simulink model "MotorLabDemonstrationV2"  (R2022b)
settings: Solver=FixedStepAuto  StartTime=0.0  StopTime=Inf  RelTol=1e-3  EnableMultiTasking=on
libraries: arduinolib x10, arduinosensorlib x2
settings Model: SimulationMode=external  ExtModeTrigDuration=2  Creator=amanc  LastModifiedBy=amanc
settings SolverCC: AutoInsertRateTranBlk=on
settings OptimizationCC: EnhancedBackFolding=on  PassReuseOutputArgsAs=Individual arguments  ZeroExternalMemoryAtStartup=off  ZeroInternalMemoryAtStartup=off  MaxStackSize=64  OptimizeBlockOrder=speed  DifferentSizesBufferReuse=on  OptimizationCustomize=off  EfficientTunableParamExpr=on
settings DebuggingCC: ParameterTunabilityLossMsg=error
settings HardwareCC: ProdBitPerInt=16  ProdBitPerPointer=16  ProdBitPerSizeT=16  ProdBitPerPtrDiffT=16  ProdLargestAtomicFloat=None  ProdWordSize=8  ProdHWDeviceType=Atmel->AVR  UseEmbeddedCoderFeatures=off
settings SFSimCC: MATLABDynamicMemAlloc=off
settings RTWCC: Description=Embedded Coder  SystemTargetFile=ert.tlc  HardwareBoard=Arduino Mega 2560  TemplateMakefile=ert_default_tmf  Toolchain=Arduino AVR  BuildConfiguration=Faster Runs
settings CodeAppCC: ForceParamTrailComments=on  OperatorAnnotations=on  SimulinkDataObjDesc=on  SFDataObjDesc=on  InsertBlockDesc=on
settings ERTTargetCC: SupportContinuousTime=on  SupportNonInlinedSFcns=on  SupportVariableSizeSignals=on  ExtMode=on  ExtModeTransport=3  ExtModeStaticAlloc=on  ExtModeAutomaticAllocSize=off  ExtModeStaticAllocSize=2048  ExtModeMexFile=ext_xcp  ExtModeMexArgs=0 3 921600  ExtModeIntrfLevel=Level2 - Open  ERTSrcFileBannerTemplate=codertarget_code_template.cgt  ERTHdrFileBannerTemplate=codertarget_code_template.cgt  ERTDataSrcFileTemplate=codertarget_code_template.cgt  ERTDataHdrFileTemplate=codertarget_code_template.cgt

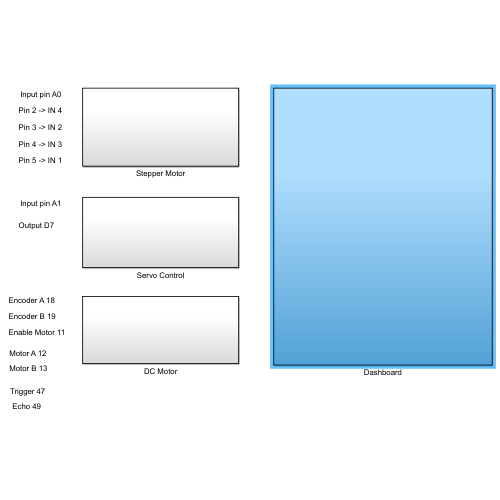
[thumbnail: Simulink's stored preview of the top-level diagram]
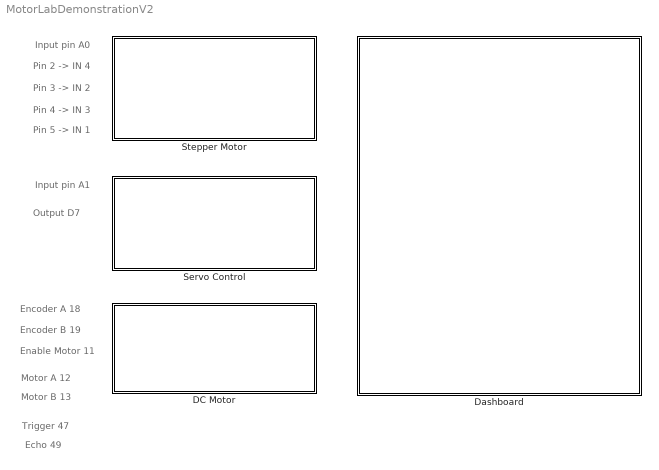
== system MotorLabDemonstrationV2 ==
  note: Echo 49
  note: Trigger 47
  note: Motor A 12
  note: Encoder A 18
  note: Pin 2 -> IN 4
  note: Input pin A0
  note: Pin 3 -> IN 2
  note: Pin 4 -> IN 3
  note: Pin 5 -> IN 1
  note: Output D7
  note: Input pin A1
  note: Encoder B 19
  note: Enable Motor 11
  note: Motor B 13
  DC Motor : Subsystem
  Dashboard : Subsystem
  Servo Control : Subsystem
  Stepper Motor : Subsystem

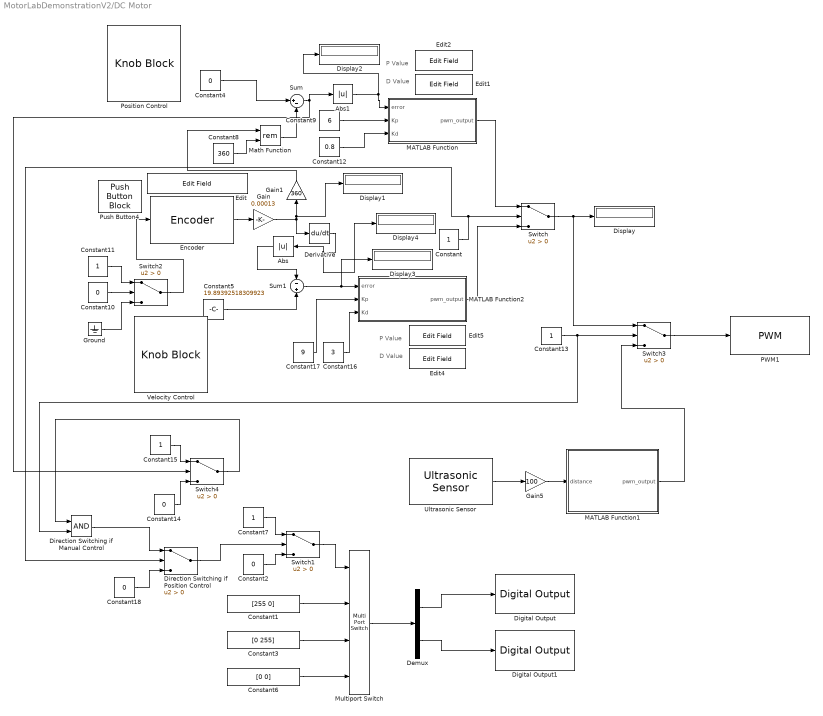
== system MotorLabDemonstrationV2/DC Motor ==
  note: P Value
  note: D Value
  note: P Value
  note: D Value
  Abs : Abs  SaturateOnIntegerOverflow=off
  Abs1 : Abs  SaturateOnIntegerOverflow=off
  Constant{,7,11,13,15} (5 alike) : Constant
  Constant1 : Constant  Value=[255 0]  OutDataTypeStr=uint8
  Constant{2,4,10,14,18} (5 alike) : Constant  Value=0
  Constant12 : Constant  Value=0.8
  Constant16 : Constant  Value=3
  Constant17 : Constant  Value=9
  Constant3 : Constant  Value=[0 255]  OutDataTypeStr=uint8
  Constant5 : Constant  Value=19.89392518309923
  Constant6 : Constant  Value=[0 0]  OutDataTypeStr=uint8
  Constant8 : Constant  Value=360
  Constant9 : Constant  Value=6
  Demux : Demux  Outputs=2
  Derivative : Derivative
  Digital Output : arduinolib/Digital Output  pinNumber=12  Direction=output  blockPlatform=arduino
  Digital Output1 : arduinolib/Digital Output  pinNumber=13  Direction=output  blockPlatform=arduino
  Direction Switching if Manual Control : Logic  AllPortsSameDT=off  OutDataTypeStr=boolean
  Direction Switching if Position Control : Switch  Criteria=u2 > Threshold  SaturateOnIntegerOverflow=off  InputSameDT=off
  Display{,1..4} (5 alike) : Display
  Edit{,1..2,4..5} (5 alike) : EditField  LabelPosition=Hide  ShowInitialText=on  Alignment=Center
  Encoder : arduinosensorlib/Encoder  InputA=18  InputB=19  Mode=Reset by external signal  SampleTime=-1
  Gain : Gain  Gain=0.00013  OutDataTypeStr=double
  Gain1 : Gain  Gain=360
  Gain5 : Gain  Gain=100
  Ground : Ground
  MATLAB Function : MATLAB Function  TreatAsAtomicUnit=on
  MATLAB Function1 : MATLAB Function  TreatAsAtomicUnit=on
  MATLAB Function2 : MATLAB Function  TreatAsAtomicUnit=on
  Math Function : Math  Operator=rem
  Multiport Switch : MultiPortSwitch  DataPortOrder=Zero-based contiguous  Inputs=2  DataPortForDefault=Additional data port  DiagnosticForDefault=None  zeroidx=on  SaturateOnIntegerOverflow=off
  PWM1 : arduinolib/PWM  pinNumber=11  frequencyType=Default  desiredFrequency=490.2  achievableFrequency=490.2
  Position Control : KnobBlock  LabelPosition=Hide  ScaleMax=360
  Push Button4 : PushButtonBlock  ButtonText=Reset  OffValue=0.000000
  Sum : Sum  Inputs=|+-
  Sum1 : Sum  Inputs=-|+
  Switch{,1..4} (5 alike) : Switch  Criteria=u2 > Threshold  SaturateOnIntegerOverflow=off  InputSameDT=off
  Ultrasonic Sensor : arduinosensorlib/Ultrasonic Sensor  NumSignalPins=2  TrigPin=47  EchoPin=49  SignalPin=3  SampleTime_=0.01  blockPlatform=ARDUINO
  Velocity Control : KnobBlock  LabelPosition=Hide  ScaleMax=20
  wires:
  Constant13/1 -> Direction Switching if Manual Control/2, Switch3/2
  MATLAB Function1/1(pwm_output) -> Switch3/3
  Constant10/1 -> Switch2/2
  Math Function/1 -> Sum/2
  Constant15/1 -> Switch4/1
  Constant11/1 -> Switch2/1
  MATLAB Function/1(pwm_output) -> Switch/1
  Gain/1 -> Display1/1, Gain1/1, Derivative/1
  MATLAB Function2/1(pwm_output) -> Switch/3
  Constant2/1 -> Switch1/3
  Gain1/1 -> Math Function/1
  Ground/1 -> Switch2/3
  Switch/1 -> Switch3/1, Display/1
  Constant17/1 -> MATLAB Function2/2(Kp)
  Sum1/1 -> Display3/1, MATLAB Function2/1(error)
  Constant12/1 -> MATLAB Function/3(Kd)
  Switch4/1 -> Direction Switching if Manual Control/1
  Constant9/1 -> MATLAB Function/2(Kp)
  Constant8/1 -> Math Function/2
  Constant5/1 -> Sum1/2
  Constant4/1 -> Sum/1
  Gain5/1 -> MATLAB Function1/1(distance)
  Constant7/1 -> Switch1/1
  Ultrasonic Sensor/1 -> Gain5/1
  Constant6/1 -> Multiport Switch/4
  Multiport Switch/1 -> Demux/1
  Constant16/1 -> MATLAB Function2/3(Kd)
  Encoder/1 -> Gain/1
  Constant1/1 -> Multiport Switch/2
  Demux/1 -> Digital Output/1
  Sum/1 -> Abs1/1, Switch4/2
  Switch1/1 -> Multiport Switch/1
  Constant14/1 -> Switch4/3
  Switch2/1 -> Encoder/1
  Constant3/1 -> Multiport Switch/3
  Constant/1 -> Direction Switching if Position Control/2, Switch/2
  Switch3/1 -> PWM1/1
  Demux/2 -> Digital Output1/1
  Constant18/1 -> Direction Switching if Position Control/3
  Direction Switching if Position Control/1 -> Switch1/2
  Direction Switching if Manual Control/1 -> Direction Switching if Position Control/1
  Derivative/1 -> Abs/1, Display4/1
  Abs/1 -> Sum1/1
  Abs1/1 -> MATLAB Function/1(error), Display2/1

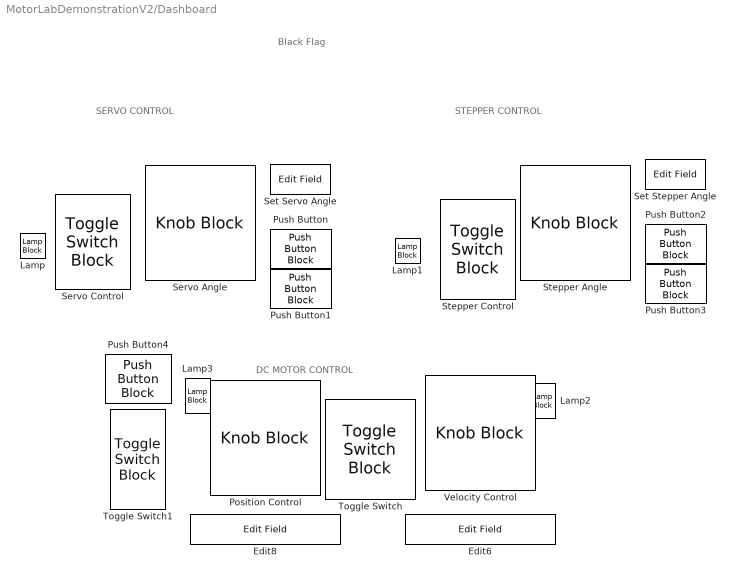
== system MotorLabDemonstrationV2/Dashboard ==
  note: Black Flag
  note: SERVO CONTROL
  note: STEPPER CONTROL
  note: DC MOTOR CONTROL
  Edit6 : EditField  LabelPosition=Hide  ShowInitialText=on  Alignment=Center
  Edit8 : EditField  LabelPosition=Hide  ShowInitialText=on  Alignment=Center
  Lamp{,1..3} (4 alike) : LampBlock  LabelPosition=Hide
  Position Control : KnobBlock  LabelPosition=Hide  ScaleMax=360
  Push Button : PushButtonBlock  ButtonText=Minimum  OnValue=0  ButtonType=Latch  OffValue=180.000000
  Push Button1 : PushButtonBlock  ButtonText=Maximum  OnValue=180  ButtonType=Latch  OffValue=0.000000
  Push Button2 : PushButtonBlock  ButtonText=Minimum  OnValue=-360  ButtonType=Latch  OffValue=0.000000
  Push Button3 : PushButtonBlock  ButtonText=Maximum  OnValue=360  ButtonType=Latch  OffValue=-360.000000
  Push Button4 : PushButtonBlock  ButtonText=Reset  OffValue=0.000000
  Servo Angle : KnobBlock  LabelPosition=Hide  ScaleMax=180
  Servo Control : ToggleSwitchBlock  LabelPosition=Hide
      settings: Values={{'Manual', 'Sensor Input'}, [0 1]}
  Set Servo Angle : EditField  LabelPosition=Hide  ShowInitialText=on  Alignment=Center
  Set Stepper Angle : EditField  LabelPosition=Hide  ShowInitialText=on  Alignment=Center
  Stepper Angle : KnobBlock  LabelPosition=Hide  ScaleMin=-360  ScaleMax=360
  Stepper Control : ToggleSwitchBlock  LabelPosition=Hide
      settings: Values={{'Manual', 'Sensor Control'}, [0 1]}
  Toggle Switch : ToggleSwitchBlock  LabelPosition=Hide
      settings: Values={{'Velocity Control', 'Position Control'}, [0 1]}
  Toggle Switch1 : ToggleSwitchBlock  LabelPosition=Hide
      settings: Values={{'Sensor', 'Manual'}, [0 1]}
  Velocity Control : KnobBlock  LabelPosition=Hide  ScaleMax=20

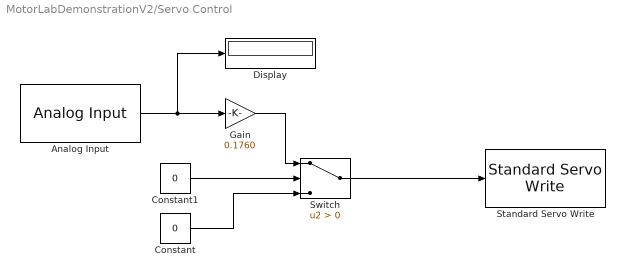
== system MotorLabDemonstrationV2/Servo Control ==
  Analog Input : arduinolib/Analog Input  pinNumber=2  ReadResultsOnly=off  ConversionTriggerSource=Software  ExternalTriggerType=uint32( 0 )  OutputDataType=uint16  EnableConversionCompleteNotify=off  EnableOuputStatus=off  SampleTime=0.01  blockPlatform=arduino
  Constant : Constant  Value=0  OutDataTypeStr=uint8
  Constant1 : Constant  Value=0
  Display : Display
  Gain : Gain  Gain=0.1760  OutDataTypeStr=uint8
  Standard Servo Write : arduinolib/Standard Servo Write  pinNumber=7  ServoIndex=0  blockPlatform=ARDUINO
  Switch : Switch  Criteria=u2 > Threshold  OutDataTypeStr=uint8  SaturateOnIntegerOverflow=off  InputSameDT=off
  wires:
  Analog Input/1 -> Display/1, Gain/1
  Constant1/1 -> Switch/2
  Switch/1 -> Standard Servo Write/1
  Gain/1 -> Switch/1
  Constant/1 -> Switch/3

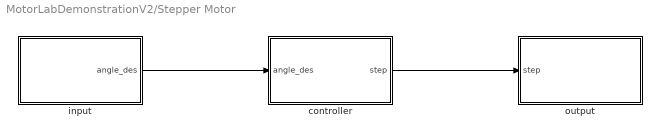
== system MotorLabDemonstrationV2/Stepper Motor ==
  controller : Subsystem
  input : Subsystem
  output : Subsystem
  wires:
  input/1(angle_des) -> controller/1(angle_des)
  controller/1(step) -> output/1(step)

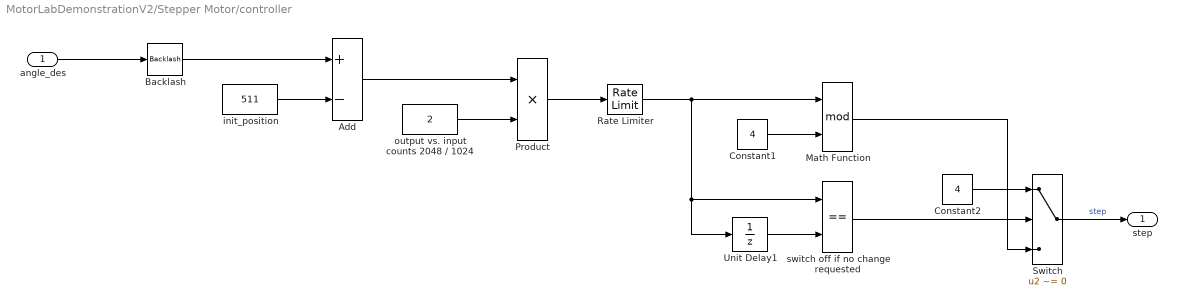
== system MotorLabDemonstrationV2/Stepper Motor/controller ==
  angle_des : Inport
  Add : Sum  Inputs=+-  InputSameDT=on
  Backlash : Backlash  BacklashWidth=6  InitialOutput=511
  Constant1 : Constant  Value=4  OutDataTypeStr=int16
  Constant2 : Constant  Value=4  OutDataTypeStr=int16
  Math Function : Math  Operator=mod  SignedPower=on  OutputSignalType=real
  Product : Product  InputSameDT=on  OutDataTypeStr=int16  RndMeth=Zero
  Rate Limiter : RateLimiter  RisingSlewLimit=100  FallingSlewLimit=-100  SampleTimeMode=inherited
  Switch : Switch  Criteria=u2 ~= 0  SaturateOnIntegerOverflow=off
  Unit Delay1 : UnitDelay  SampleTime=-1  HasFrameUpgradeWarning=on
  init_position : Constant  Value=511  OutDataTypeStr=int16
  output vs. input counts 2048 / 1024 : Constant  Value=2  OutDataTypeStr=int16
  switch off if no change requested : RelationalOperator  Operator===  OutDataTypeStr=boolean
  step : Outport
  wires:
  angle_des/1 -> Backlash/1
  init_position/1 -> Add/2
  Add/1 -> Product/1
  output vs. input counts 2048 / 1024/1 -> Product/2
  Product/1 -> Rate Limiter/1
  Constant1/1 -> Math Function/2
  Rate Limiter/1 -> switch off if no change requested/1, Unit Delay1/1, Math Function/1
  Backlash/1 -> Add/1
  Switch/1 -> step/1  "step"
  Constant2/1 -> Switch/1
  switch off if no change requested/1 -> Switch/2
  Math Function/1 -> Switch/3
  Unit Delay1/1 -> switch off if no change requested/2

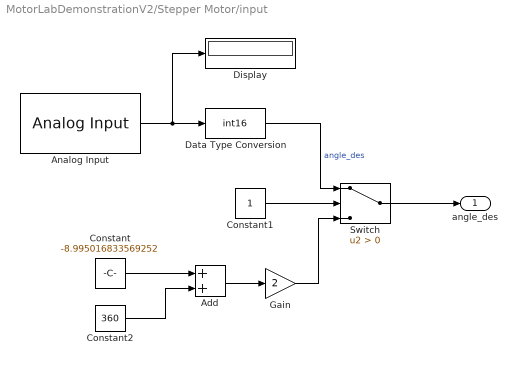
== system MotorLabDemonstrationV2/Stepper Motor/input ==
  Add : Sum
  Analog Input : arduinolib/Analog Input  pinNumber=0  ReadResultsOnly=off  ConversionTriggerSource=Software  ExternalTriggerType=uint32( 0 )  OutputDataType=uint16  EnableConversionCompleteNotify=off  EnableOuputStatus=off  SampleTime=0.010  blockPlatform=arduino
  Constant : Constant  Value=-8.995016833569252
  Constant1 : Constant  OutDataTypeStr=int16
  Constant2 : Constant  Value=360  OutDataTypeStr=int16
  Data Type Conversion : DataTypeConversion  OutDataTypeStr=int16  SaturateOnIntegerOverflow=off  RndMeth=Floor
  Display : Display
  Gain : Gain  Gain=2
  Switch : Switch  Criteria=u2 > Threshold  OutDataTypeStr=int16  SaturateOnIntegerOverflow=off  InputSameDT=off
  angle_des : Outport
  wires:
  Analog Input/1 -> Display/1, Data Type Conversion/1
  Switch/1 -> angle_des/1
  Data Type Conversion/1 -> Switch/1  "angle_des"
  Constant1/1 -> Switch/2
  Gain/1 -> Switch/3
  Add/1 -> Gain/1
  Constant/1 -> Add/1
  Constant2/1 -> Add/2

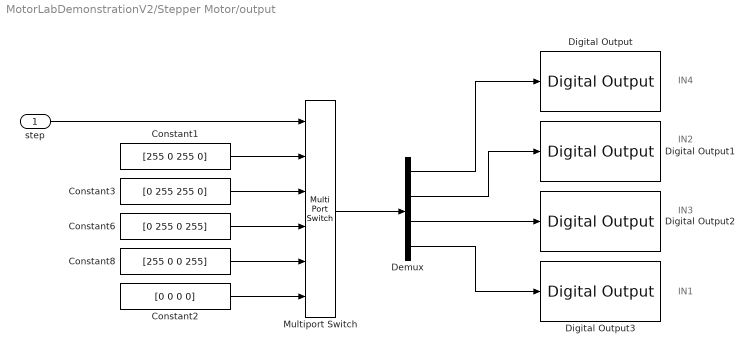
== system MotorLabDemonstrationV2/Stepper Motor/output ==
  note: IN4
  note: IN2
  note: IN3
  note: IN1
  step : Inport
  Constant1 : Constant  Value=[255 0 255 0]  OutDataTypeStr=uint8
  Constant2 : Constant  Value=[0 0 0 0]  OutDataTypeStr=uint8
  Constant3 : Constant  Value=[0 255 255 0]  OutDataTypeStr=uint8
  Constant6 : Constant  Value=[0 255 0 255]  OutDataTypeStr=uint8
  Constant8 : Constant  Value=[255 0 0 255]  OutDataTypeStr=uint8
  Demux : Demux
  Digital Output : arduinolib/Digital Output  pinNumber=2  Direction=output  blockPlatform=arduino
  Digital Output1 : arduinolib/Digital Output  pinNumber=3  Direction=output  blockPlatform=arduino
  Digital Output2 : arduinolib/Digital Output  pinNumber=4  Direction=output  blockPlatform=arduino
  Digital Output3 : arduinolib/Digital Output  pinNumber=5  Direction=output  blockPlatform=arduino
  Multiport Switch : MultiPortSwitch  DataPortOrder=Zero-based contiguous  Inputs=4  DataPortForDefault=Additional data port  DiagnosticForDefault=None  zeroidx=on  SaturateOnIntegerOverflow=off
  wires:
  Demux/1 -> Digital Output/1
  Demux/2 -> Digital Output1/1
  Demux/3 -> Digital Output2/1
  Demux/4 -> Digital Output3/1
  Constant1/1 -> Multiport Switch/2
  Multiport Switch/1 -> Demux/1
  step/1 -> Multiport Switch/1
  Constant3/1 -> Multiport Switch/3
  Constant6/1 -> Multiport Switch/4
  Constant8/1 -> Multiport Switch/5
  Constant2/1 -> Multiport Switch/6

== matlab function MotorLabDemonstrationV2/DC Motor/MATLAB Function1 ==
  data: distance input; pwm_output output
function pwm_output = map_distance_to_pwm(distance)
    % Map distance to range 0 to 1
    distance_min = 3;
    distance_max = 25;
    pwm_min = 0;
    pwm_max = 255;
    distance_normalized = (distance - distance_min) / (distance_max - distance_min);
    
    % Map distance to range pwm_min to pwm_max
    pwm_output = round(distance_normalized * (pwm_max - pwm_min) + pwm_min);
    
    % Limit PWM output to specified range
    pwm_output = min(max(pwm_output, pwm_min), pwm_max);
end

== matlab function MotorLabDemonstrationV2/DC Motor/MATLAB Function ==
  data: error input; pwm_output output; Kp input; Kd input

function pwm_output = pid_controller_angle(error, Kp,Kd)
    persistent last_error;
    % Calculate proportional term
    if isempty(last_error)
        last_error = 0;
    end
    proportional_term = Kp * error;
    derivative_term = Kd * (error - last_error);
   
    % Calculate total control signal
    control_signal = proportional_term + derivative_term;
    
    % Map control signal to PWM output range
    pwm_output = round((control_signal / 180) * 255);
    
    % Limit PWM output to specified range
    pwm_output = min(max(pwm_output, 0), 255);
    last_error = error;
end

== matlab function MotorLabDemonstrationV2/DC Motor/MATLAB Function2 ==
  data: error input; pwm_output output; Kp input; Kd input

function pwm_output = pid_controller_velocity(error, Kp,Kd)
    persistent last_error_vel;
    % Calculate proportional term
    if isempty(last_error_vel)
        last_error_vel = 0;
    end
    proportional_term = Kp * error;
    derivative_term = Kd * (error - last_error_vel);
   
    % Calculate total control signal
    control_signal = proportional_term + derivative_term;
    
    % Map control signal to PWM output range
    pwm_output = round((control_signal / 180) * 255);
    
    % Limit PWM output to specified range
    pwm_output = min(max(pwm_output, 0), 255);
    last_error_vel = error;
end
